simulink model "Electromech_sys_linearized_obs"  (R2025b)
settings: Solver=VariableStepAuto  StartTime=0.0  StopTime=28  RelTol=1e-3
values from neighbouring files (symbols this model uses):
  A = (J - R) * Hxx    [linearize_electromech.m]    (also in linearize_mech.m = (J - R) * Hxx + grad_g * u_eq_mech)
  B = g    [linearize_electromech.m]    (also in linearize_mech.m)
  C = g' * Hxx    [linearize_electromech.m]    (also in linearize_mech.m = g.' * Hxx + gradH.' * grad_g)
  p_0 = 0    [Init_Simulink_param_lin_Electromech.m]
  ptilde_0 = phat_0 - x_eq(2)    [Init_Simulink_param_lin_Electromech.m]
  q_0 = 0    [Init_Simulink_param_lin_Electromech.m]
  Q_0 = 0    [Init_Simulink_param_lin_Electromech.m]
  qtilde_0 = qhat_0 - x_eq(1)    [Init_Simulink_param_lin_Electromech.m]
  Qtilde_0 = Qhat_0 - x_eq(3)    [Init_Simulink_param_lin_Electromech.m]
  x_eq = [q_eq; p_eq; Q_eq]    [equilibrium_electromech.m]
  y_eq = (Q_eq) / (re * epsllon * (q_eq + q0)^4)    [equilibrium_electromech.m]
undefined symbols (not defined in the file or in its folder): params, u_eq
libraries: simulink x1
settings Model: Creator=filippougolini  LastModifiedBy=filippougolini

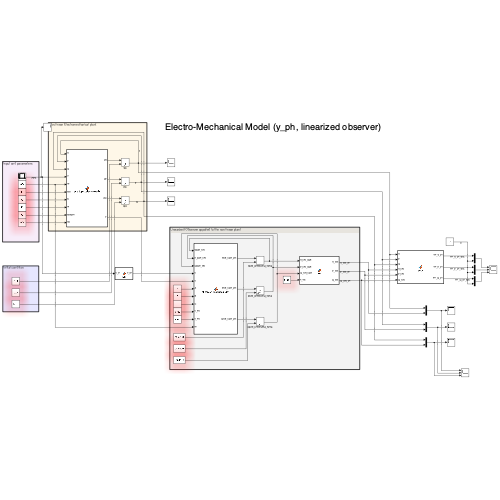
[thumbnail: Simulink's stored preview of the top-level diagram]
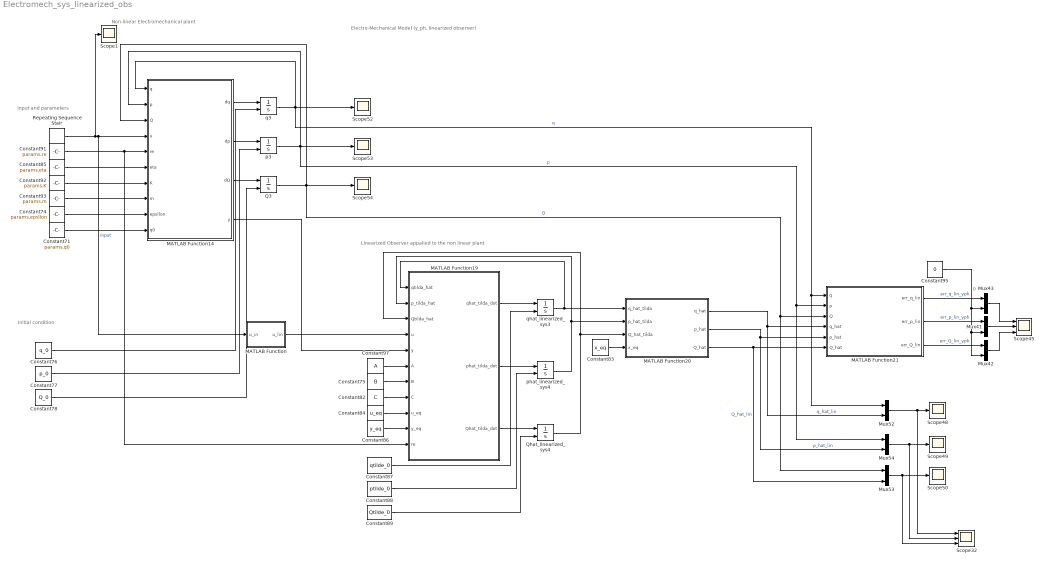
== system Electromech_sys_linearized_obs ==
  note: Initial condition
  note: Input and parameters
  note: Electro-Mechanical Model (y_ph, linearized observer)
  note: Non-linear Electromechanical plant
  note: Linearized Observer appalied to the non linear plant
  Constant71 : Constant  Value=params.q0
  Constant74 : Constant  Value=params.epsllon
  Constant75 : Constant  Value=B
  Constant76 : Constant  Value=q_0
  Constant77 : Constant  Value=p_0
  Constant78 : Constant  Value=Q_0
  Constant82 : Constant  Value=C
  Constant83 : Constant  Value=x_eq
  Constant84 : Constant  Value=u_eq
  Constant85 : Constant  Value=params.eta
  Constant86 : Constant  Value=y_eq
  Constant87 : Constant  Value=qtilde_0
  Constant88 : Constant  Value=ptilde_0
  Constant89 : Constant  Value=Qtilde_0
  Constant91 : Constant  Value=params.re
  Constant92 : Constant  Value=params.K
  Constant93 : Constant  Value=params.m
  Constant95 : Constant  Value=0
  Constant97 : Constant  Value=A
  MATLAB Function : MATLAB Function  TreatAsAtomicUnit=on
  MATLAB Function14 : MATLAB Function  TreatAsAtomicUnit=on
  MATLAB Function19 : MATLAB Function  TreatAsAtomicUnit=on
  MATLAB Function20 : MATLAB Function  TreatAsAtomicUnit=on
  MATLAB Function21 : MATLAB Function  TreatAsAtomicUnit=on
  Mux{41..43,52..54} (6 alike) : Mux  Inputs=2
  Q3 : Integrator  InitialConditionSource=external
  Qhat_linearized_sys4 : Integrator  InitialConditionSource=external  InitialCondition=20e-5
  Repeating Sequence Stair : simulink/Sources/Repeating Sequence Stair  OutValues=[0 4.9e3 5e3 4.8e3 5.1e3 5e3 0].'  tsamp=4  OutMin=[]  OutMax=[]  OutDataTypeStr=double  OutputDataTypeScalingMode=double  OutDataType=fixdt(0,8)  ConRadixGroup=Best Precision: Vector-wise  OutScaling=2^-12
  Scope{1,48..50,52..54} (7 alike) : Scope
      Scope1 settings: ActiveDisplayYMinimum=-637.49999999999989  ActiveDisplayYMaximum=5737.5
      Scope48 settings: ActiveDisplayYMinimum=-0.005346473589274754  ActiveDisplayYMaximum=0.00095804165769468883  DataLoggingVariableName=ScopeData48
      Scope49 settings: ActiveDisplayYMinimum=-0.0045902088543352884  ActiveDisplayYMaximum=0.00516486271210546  DataLoggingVariableName=ScopeData49
      Scope50 settings: ActiveDisplayYMinimum=-2.096197823231283E-8  ActiveDisplayYMaximum=1.8865780409081551E-7  DataLoggingVariableName=ScopeData50
      Scope52 settings: ActiveDisplayYMinimum=-4.0944874698701246E-5  ActiveDisplayYMaximum=0.0003685038722883113  DataLoggingVariableName=ScopeData52
      Scope53 settings: ActiveDisplayYMinimum=-1  ActiveDisplayYMaximum=1  DataLoggingVariableName=ScopeData53
      Scope54 settings: ActiveDisplayYMinimum=-1  ActiveDisplayYMaximum=1  DataLoggingVariableName=ScopeData54
  Scope32 : Scope  NumInputPorts=3
      settings: ActiveDisplayString=3  ActiveDisplayYMinimum=-7.2477560286155934E-9  ActiveDisplayYMaximum=5.8972418888280151E-8  DataLoggingVariableName=ScopeData32
  Scope45 : Scope  NumInputPorts=3
      settings: ActiveDisplayYMinimum=-2.023476500793105E-6  ActiveDisplayYMaximum=1.2609150425400225E-5  DataLoggingVariableName=ScopeData45
  p3 : Integrator  InitialConditionSource=external
  phat_linearized_sys4 : Integrator  InitialConditionSource=external  InitialCondition=20e-5
  q3 : Integrator  InitialConditionSource=external
  qhat_linearized_sys3 : Integrator  InitialConditionSource=external  InitialCondition=20e-5
  wires:
  MATLAB Function14/2(dp) -> p3/1
  Constant92/1 -> MATLAB Function14/7(K)
  Constant91/1 -> MATLAB Function19/11(re), MATLAB Function14/5(re)
  Constant74/1 -> MATLAB Function14/9(epsllon)
  Constant85/1 -> MATLAB Function14/6(eta)
  Constant76/1 -> q3/2
  Constant93/1 -> MATLAB Function14/8(m)
  Constant78/1 -> Q3/2
  Constant71/1 -> MATLAB Function14/10(q0)
  MATLAB Function14/3(dQ) -> Q3/1
  MATLAB Function14/1(dq) -> q3/1
  Constant77/1 -> p3/2
  Constant84/1 -> MATLAB Function19/9(u_eq)
  MATLAB Function19/1(qhat_tilda_dot) -> qhat_linearized_sys3/1
  MATLAB Function19/3(Qhat_tilda_dot) -> Qhat_linearized_sys4/1
  Constant87/1 -> qhat_linearized_sys3/2
  MATLAB Function14/4(y) -> MATLAB Function19/5(y)
  Mux43/1 -> Scope45/1
  Constant95/1 -> Mux42/2, Mux41/2, Mux43/2  "0"
  Constant97/1 -> MATLAB Function19/6(A)
  Constant88/1 -> phat_linearized_sys4/2
  q3/1 -> MATLAB Function14/1(q), Mux52/1, MATLAB Function21/1(q), Scope52/1  "q"
  Q3/1 -> MATLAB Function14/3(Q), Mux53/1, MATLAB Function21/3(Q), Scope54/1  "Q"
  Qhat_linearized_sys4/1 -> MATLAB Function19/3(Qtilda_hat), MATLAB Function20/3(Q_hat_tilda)
  Repeating Sequence Stair/1 -> Scope1/1, MATLAB Function/1(u_in), MATLAB Function14/4(u)  "input"
  qhat_linearized_sys3/1 -> MATLAB Function20/1(q_hat_tilda), MATLAB Function19/1(qtilda_hat)
  p3/1 -> MATLAB Function14/2(p), Mux54/1, MATLAB Function21/2(p), Scope53/1  "p"
  Constant86/1 -> MATLAB Function19/10(y_eq)
  Constant83/1 -> MATLAB Function20/4(x_eq)
  MATLAB Function21/3(err_Q_lin) -> Mux42/1  "err_Q_lin_yph"
  Mux52/1 -> Scope32/1, Scope48/1
  Constant75/1 -> MATLAB Function19/7(B)
  MATLAB Function21/1(err_q_lin) -> Mux43/1  "err_q_lin_yph"
  Constant82/1 -> MATLAB Function19/8(C)
  Mux54/1 -> Scope32/2, Scope49/1
  MATLAB Function19/2(phat_tilda_dot) -> phat_linearized_sys4/1
  Constant89/1 -> Qhat_linearized_sys4/2
  Mux42/1 -> Scope45/3
  phat_linearized_sys4/1 -> MATLAB Function19/2(p_tilda_hat), MATLAB Function20/2(p_hat_tilda)
  Mux53/1 -> Scope32/3, Scope50/1
  MATLAB Function21/2(err_p_lin) -> Mux41/1  "err_p_lin_yph"
  Mux41/1 -> Scope45/2
  MATLAB Function20/1(q_hat) -> Mux52/2, MATLAB Function21/4(q_hat)  "q_hat_lin"
  MATLAB Function20/2(p_hat) -> Mux54/2, MATLAB Function21/5(p_hat)  "p_hat_lin"
  MATLAB Function20/3(Q_hat) -> Mux53/2, MATLAB Function21/6(Q_hat)  "Q_hat_lin"
  MATLAB Function/1(u_lin) -> MATLAB Function19/4(u)

== matlab function Electromech_sys_linearized_obs/MATLAB Function20 ==
  data: q_hat_tilda input; p_hat_tilda input; Q_hat_tilda input; x_eq input; q_hat output; p_hat output; Q_hat output
function [q_hat, p_hat, Q_hat] = fcn(q_hat_tilda, p_hat_tilda, Q_hat_tilda, ...
    x_eq)
    
    q_tilda_eq = x_eq(1);
    p_tilda_eq = x_eq(2);
    Q_tilda_eq = x_eq(3);

    
    
    q_hat = q_hat_tilda + q_tilda_eq;
    p_hat = p_hat_tilda + p_tilda_eq;
    Q_hat = Q_hat_tilda + Q_tilda_eq;
end

== matlab function Electromech_sys_linearized_obs/MATLAB Function21 ==
  data: q input; err_q_lin output; p input; Q input; q_hat input; p_hat input; Q_hat input; err_p_lin output; err_Q_lin output
function [err_q_lin, err_p_lin, err_Q_lin] = error(q, p, Q, q_hat, p_hat, Q_hat)

    err_q_lin = q - q_hat;
    err_p_lin = p - p_hat;
    err_Q_lin = Q - Q_hat;
end

== matlab function Electromech_sys_linearized_obs/MATLAB Function ==
  data: u_in input; u_lin output
function u_lin = fcn(u_in)

u_lin = u_in;

== matlab function Electromech_sys_linearized_obs/MATLAB Function14 ==
  data: q input; p input; Q input; u input; dq output; re input; eta input; K input; m input; epsllon input; q0 input; dp output; dQ output; y output
function [dq, dp, dQ, y] = plant_pH_electromech(q, p, Q, u, re, eta, K, m, epsllon, q0)
% Electro-mechanical pH plant

    % Parameters: m, K, eta, eps, re, q0 in workspace

    J = [  0  1  0;
          -1  0  0;
           0  0  0 ];

    R = diag([0, eta, 1/re]);
    g = [0; 0; 1/re];

    % Hamiltonian gradient gradH(q,p,Q)
    Cq   = epsllon * (q + q0)^4;

    dHdq = K*q - 2*Q^2 / (epsllon * (q + q0)^5);
    dHdp = p / m;
    dHdQ = Q / Cq;

    gradH = [dHdq; dHdp; dHdQ];

    xdot = (J - R) * gradH + g*u;

    y = Q / (re * epsllon * (q + q0)^4);

    
    dq = xdot(1);
    dp = xdot(2);
    dQ = xdot(3);
end

== matlab function Electromech_sys_linearized_obs/MATLAB Function19 ==
  data: qhat_tilda_dot output; phat_tilda_dot output; Qhat_tilda_dot output; qtilda_hat input; p_tilda_hat input; Qtilda_hat input; u input; y input; A input; B input; C input; u_eq input; y_eq input; re input
function [qhat_tilda_dot, phat_tilda_dot, Qhat_tilda_dot] = ...
    observer_linearized_dev(qtilda_hat, p_tilda_hat, Qtilda_hat, u, y, A, ...
    B, C, u_eq, y_eq, re)

    % ---- Deviation state and absolute estimate ---- 
    delta_xhat = [qtilda_hat; p_tilda_hat; Qtilda_hat]; % 3x1 
    % ---- Deviation input and output ---- 
    delta_u = u - u_eq; 
    delta_y = y - y_eq;

    g = [0; 0; 1/re];
    gamma = 20;
    L  = gamma * g;

    delta_xhatdot = A*delta_xhat + B*delta_u + L' * (delta_y - C'*delta_xhat);

    % ---- Derivatives of deviation states ---- 
    qhat_tilda_dot = delta_xhatdot(1); 
    phat_tilda_dot = delta_xhatdot(2); 
    Qhat_tilda_dot = delta_xhatdot(3);
end
